simulink model "demo"  (R2024b)
settings: Solver=ode3  StartTime=0.0  StopTime=1.0  FixedStep=.01  RelTol=1e-3  EnableMultiTasking=on
model workspace (MAT data in the model file):
  F = [47.5030304796; 46.9110614304; 47.028984707; 45.6862216169; 44.6182372756; 0]
  FR = [-46.5418915863 -46.5418915863 -46.5418915863 -46.5418915863 -46.5418915863 -46.5418915863 -46.5418915863 -46.5418915863 -46.5418915863 -46.5418915863 -46.5418915863 -46.5418915863 ... (901 elements, 1x901)]
  InputSize = 6
  M = [13.6965475483 27.5033300826 -29.1231309962 -36.2545983973 -28.5352204611 23.5897220685 -14.907640199 1.71607773467 -6.59423100681 35.1253819893 -6.10963272822 7.71481328081 ... (3003 elements, 1001x3)]
  N = 24
  T : table (value not decoded)
  TimeSteps = 101
  X = [-5960.81977319 232.260971899 -1604.51423784 -5520.60108545 -9468.97440908 -5944.7629474 -8448.78266584 256.487426718 -8675.78613889 4363.6350641 -9034.85038905 -325.411444222 ... (16 elements, 1x16)]
  a1 = -5.99281334265
  a2 = 6.7586120696
  a3 = -8.48382923723
  axial = 0
  axial_change = [-31.4255261802 -30.7695758416 -31.1885211647 -29.9884626265 -30.6698057294 -31.9546590717 -31.9773114122 -31.0590125801 -31.4973929014 -31.4591407909 -31.9452553476 -31.5912458676 ... (1000 elements, 1000x1)]
  cmd : object (value not decoded)
  cs : handle (value not decoded)
  curPath = '/Users/khouloud.gaaloul/Documents/Projects/ModeTestingData/Problems'
  d = 17
  hcvdt_cmd_fcs_dps2 = [0 0 0 0 0 0 0 0 0 0 0 0 ... (1000 elements, 1000x1)]
  height = 0
  height_change = [-31.99975 -31.8 -31.8 -31.8 -31.99975 -31.8 -31.8 -31.8 -31.99975 -31.8 -31.99975 -31.8 ... (1000 elements, 1000x1)]
  hws = [3707764736; 2; 1; 1; 2; 2]
  i = 8
  j = 16
  lcvdt_cmd_fcs_dps2 = [-172.441967394 -126.914225002 101.408793207 185.523827088 35.8854623366 -8.64188069371 100.038910088 117.411213524 -22.955981386 -181.02871483 29.1905053694 73.1255676915 ... (1000 elements, 1000x1)]
  list : object (value not decoded)
  mcvdt_cmd_fcs_dps2 = [0 0 0 0 0 0 0 0 0 0 0 0 ... (1000 elements, 1000x1)]
  model_cs : handle (value not decoded)
  modelpath = '/Users/khouloud.gaaloul/Documents/Projects/Benchmark/Simulink Models/3_regulators/'
  n = 6
  nbrInputs = 16
  nbrTimeSteps = 1001
  ncvdt_cmd_fcs_dps2 = [0 0 0 0 0 0 0 0 0 0 0 0 ... (1000 elements, 1000x1)]
  pitch = 0
  pitch_change = [-29.1847957495 -33.8637964543 -47.1499761463 -47.1433778125 -41.276337879 -45.6028204159 -37.5507526458 -39.9406146771 -31.3489497461 -28.9458637417 -26.1569554928 -41.8886302088 ... (1000 elements, 1000x1)]
  req = 'R2'
  roll = 0
  roll_change = [-41.4686910833 -44.5265370434 -48.3240218587 -45.9838380142 -45.0248995082 -48.7661309065 -46.4562699575 -48.9496331544 -43.3304519808 -46.1818460958 -48.131234837 -44.5028232735 ... (1000 elements, 1000x1)]
  simOut : Simulink.SimulationOutput (value not decoded)
  t = [0 0.01 0.02 0.03 0.04 0.05 0.06 0.07 0.08 0.09 0.1 0.11 ... (101 elements, 101x1)]
  u = [-5960.81977319 232.260971899 -1604.51423784 -5520.60108545 -9468.97440908 -5944.7629474 -8448.78266584 256.487426718 -8675.78613889 4363.6350641 -9034.85038905 -325.411444222 ... (16 elements, 1x16)]
  var : object (value not decoded)
  varout = [-172.441967394 -126.914225002 101.408793207 185.523827088 35.8854623366 -8.64188069371 100.038910088 117.411213524 -22.955981386 -181.02871483 29.1905053694 73.1255676915 ... (5000 elements, 1000x5)]
  vars : object (value not decoded)
  xcvdt_cmd_fcs_dps2 = [0 0 0 0 0 0 0 0 0 0 0 0 ... (1000 elements, 1000x1)]
  yaw = 0
  yaw_change = [-49.1533965478 -48.6929062567 -47.6689253182 -47.3940427916 -49.3847503901 -46.8626914945 -44.1531478971 -48.0156975418 -49.8912914581 -49.5126245185 -48.3496741118 -48.8753270352 ... (1000 elements, 1000x1)]
undefined symbols (not defined in the file or in its folder): transition_v, transition_y
(part 2 of 2)

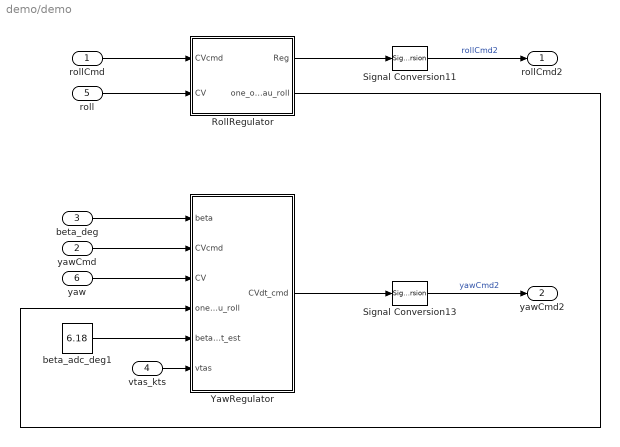
== system demo/demo ==
  "rollCmd " : Inport  OutDataTypeStr=double
  yawCmd : Inport  Port=2  OutDataTypeStr=double
  beta_deg : Inport  Port=3
  vtas_kts : Inport  Port=4
  roll : Inport  Port=5  OutDataTypeStr=double
  yaw : Inport  Port=6  OutDataTypeStr=double
  RollRegulator : Subsystem
  Signal Conversion11 : SignalConversion  ConversionOutput=Contiguous copy  OverrideOpt=on
  Signal Conversion13 : SignalConversion  ConversionOutput=Contiguous copy  OverrideOpt=on
  YawRegulator : Subsystem
  beta_adc_deg1 : Constant  Value=6.18
  rollCmd2 : Outport  VectorParamsAs1DForOutWhenUnconnected=off
  yawCmd2 : Outport  Port=2  VectorParamsAs1DForOutWhenUnconnected=off
  wires:
  beta_deg/1 -> YawRegulator/1(beta)
  vtas_kts/1 -> YawRegulator/6(vtas)
  Signal Conversion11/1 -> rollCmd2/1  "rollCmd2"
  RollRegulator/2(one_over_Tau_roll) -> YawRegulator/4(one_over_Tau_roll)
  roll/1 -> RollRegulator/2(CV)
  yaw/1 -> YawRegulator/3(CV)
  beta_adc_deg1/1 -> YawRegulator/5(beta_dot_est)
  Signal Conversion13/1 -> yawCmd2/1  "yawCmd2"
  "rollCmd "/1 -> RollRegulator/1(CVcmd)
  RollRegulator/1(Reg) -> Signal Conversion11/1
  YawRegulator/1(CVdt_cmd) -> Signal Conversion13/1
  yawCmd/1 -> YawRegulator/2(CVcmd)

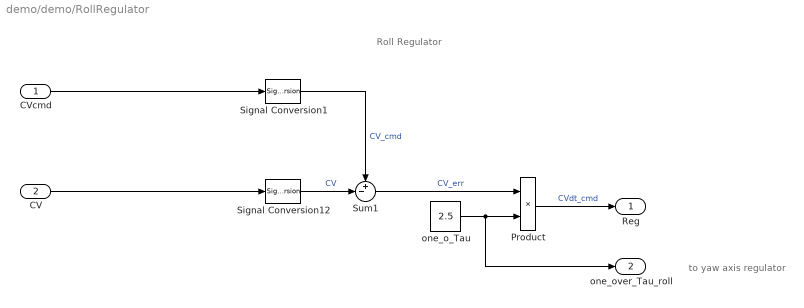
== system demo/demo/RollRegulator ==
  note: Roll Regulator
  note: to yaw axis regulator
  CVcmd : Inport
  CV : Inport  Port=2
  Product : Product  RndMeth=Zero
  Signal Conversion1 : SignalConversion  ConversionOutput=Contiguous copy  OverrideOpt=on
  Signal Conversion12 : SignalConversion  ConversionOutput=Contiguous copy  OverrideOpt=on
  Sum1 : Sum  Inputs=+-|  InputSameDT=on  SaturateOnIntegerOverflow=on  OutDataTypeStr=Inherit: Same as first input
  one_o_Tau : Constant  Value=2.5
  Reg : Outport  VectorParamsAs1DForOutWhenUnconnected=off
  one_over_Tau_roll : Outport  Port=2  VectorParamsAs1DForOutWhenUnconnected=off
  wires:
  Sum1/1 -> Product/1  "CV_err"
  Signal Conversion1/1 -> Sum1/1  "CV_cmd"
  Signal Conversion12/1 -> Sum1/2  "CV"
  CV/1 -> Signal Conversion12/1
  CVcmd/1 -> Signal Conversion1/1
  one_o_Tau/1 -> Product/2, one_over_Tau_roll/1
  Product/1 -> Reg/1  "CVdt_cmd"

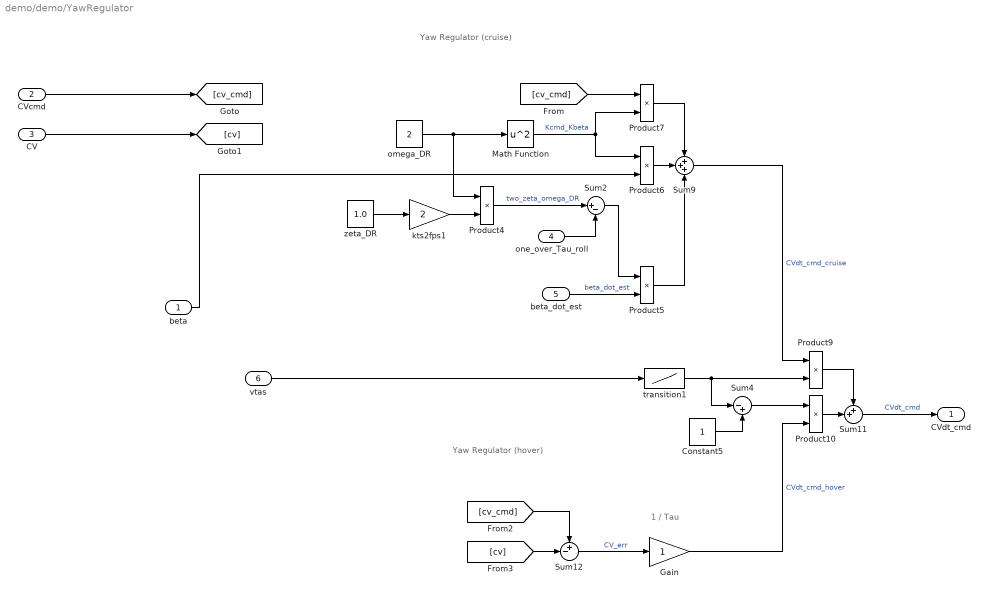
== system demo/demo/YawRegulator ==
  note: Yaw Regulator (hover)
  note: 1 / Tau
  note: Yaw Regulator (cruise)
  beta : Inport
  CVcmd : Inport  Port=2
  CV : Inport  Port=3
  one_over_Tau_roll : Inport  Port=4
  beta_dot_est : Inport  Port=5
  vtas : Inport  Port=6
  Constant5 : Constant
  Gain : Gain
  Math Function : Math  Operator=square  SignedPower=on
  Product{4..7,9..10} (6 alike) : Product  SaturateOnIntegerOverflow=on  OutDataTypeStr=Inherit: Same as first input
  Sum11 : Sum  Inputs=++|
  Sum12 : Sum  Inputs=+-|  InputSameDT=on  SaturateOnIntegerOverflow=on  OutDataTypeStr=Inherit: Same as first input
  Sum2 : Sum  Inputs=|+-  InputSameDT=on  SaturateOnIntegerOverflow=on  OutDataTypeStr=Inherit: Same as first input
  Sum4 : Sum  Inputs=|-+
  Sum9 : Sum  Inputs=+++  InputSameDT=on  SaturateOnIntegerOverflow=on  OutDataTypeStr=Inherit: Same as first input
  kts2fps1 : Gain  Gain=2
  omega_DR : Constant  Value=2
  transition1 : Lookup  InputValues=transition_v  Table=transition_y  SaturateOnIntegerOverflow=off
  zeta_DR : Constant  Value=1.0
  CVdt_cmd : Outport  VectorParamsAs1DForOutWhenUnconnected=off
  wires:
  beta/1 -> Product6/2
  Product6/1 -> Sum9/2
  omega_DR/1 -> Math Function/1, Product4/1
  Product7/1 -> Sum9/1
  Math Function/1 -> Product6/1, Product7/2  "Kcmd_Kbeta"
  Sum11/1 -> CVdt_cmd/1  "CVdt_cmd"
  transition1/1 -> Sum4/1, Product9/2
  Product9/1 -> Sum11/1
  Constant5/1 -> Sum4/2
  Sum4/1 -> Product10/1
  Product10/1 -> Sum11/2
  Sum9/1 -> Product9/1  "CVdt_cmd_cruise"
  Sum12/1 -> Gain/1  "CV_err"
  beta_dot_est/1 -> Product5/2  "beta_dot_est"
  Gain/1 -> Product10/2  "CVdt_cmd_hover"
  [cv_cmd] -> Product7/1
  [cv_cmd] -> Sum12/1
  [cv] -> Sum12/2
  zeta_DR/1 -> kts2fps1/1
  kts2fps1/1 -> Product4/2
  Product4/1 -> Sum2/1  "two_zeta_omega_DR"
  one_over_Tau_roll/1 -> Sum2/2
  Product5/1 -> Sum9/3
  Sum2/1 -> Product5/1
  vtas/1 -> transition1/1
  CVcmd/1 -> [cv_cmd]
  CV/1 -> [cv]
